simulink model "Controller_20231019"  (R2021b)
settings: Solver=ode4  StartTime=0.0  StopTime=5  FixedStep=0.01  RelTol=1e-3
values from neighbouring files (symbols this model uses):
  diag_M = diagonalize(M_frak0, M_frak)    [Initiate_KUKA_inv.m]
  iota0 = eye(6,6)    [Initiate_KUKA_inv.m]
  K_d = 10*[1.3*eye(3) zeros(3);zeros(3) 0.8*eye(3)]    [Initiate_FQ.m]    (also in Initiate_KUKA_inv.m = 5*[0.7*eye(3) zeros(3);zeros(3) 0.5*eye(3)])
  K_i = 5*[0.1*eye(3) zeros(3);zeros(3) 0.01*eye(3)]    [Initiate_FQ.m]    (also in Initiate_KUKA_inv.m = 5*[0.01*eye(3) zeros(3);zeros(3) 0.001*eye(3)])
  K_p = 100*[0.1 0 0 0 0 0;0 0.1 0 0 0 0; 0 0 0.1 0 0 0; 0 0 0 0.01 0 0 ... (first row only)    [Initiate_FQ.m]    (also in Initiate_KUKA_inv.m = 5*[0.1 0 0 0 0 0;0 0.1 0 0 0 0; 0 0 0.1 0 0 0; 0 0 0 0.01 0 )
  m0 = robot.Bodies{1,n+1}.Mass    [Initiate_KUKA_inv.m]
  M_t = (((Adjoint(g_It))'\M_t_body)/(Adjoint(g_It)))    [Initiate_FQ.m]    (also in Initiate_KUKA_inv.m = [eye(3)*mt zeros(3); zeros(3) eye(3)*80])
  mm = zeros(1,n)    [Initiate_KUKA_inv.m]
  mu = P0    [Initiate_FQ.m]    (also in Initiate_KUKA_inv.m = zeros(6,1))
  mu_t = inv((Adjoint(g_It))')*M_t_body*[V_It;w_t]    [Initiate_FQ.m]    (also in Initiate_KUKA_inv.m = M_t*[V_0t;w_t])
  q_dot_m = [0;0;0;0;0;0;0]    [Initiate_FQ.m]    (also in Initiate_KUKA_inv.m)
  q_m = [0.2;1.2;0.3;2.5;0.5;1.5;0.6]    [Initiate_FQ.m]    (also in Initiate_KUKA_inv.m = [0;0;0;0;0;0;0])
  rho_0t = [0.24;0.26;0.25]    [Initiate_KUKA_inv.m]
  sc_size = 1    [Initiate_KUKA_inv.m]
  V_0t = [-0.01;-0.01;0]    [Initiate_KUKA_inv.m]
  V_I0 = [-0.001;-0.001;0.0;-0.001;0.001;0.002]    [Initiate_FQ.m]    (also in Initiate_KUKA_inv.m = [0;0;0;0;0;0])
  Xi_m_matrix = zeros(6*n,n)    [Initiate_KUKA_inv.m]
undefined symbols (not defined in the file or in its folder): I0, Ie, Im, me, X, Xi_m, Y, Z
libraries: nesl_utility x83, sm_lib x78, robotcorelib x4
(part 1 of 4)
settings Model: Creator=Bmmog  LastModifiedBy=Bmmog

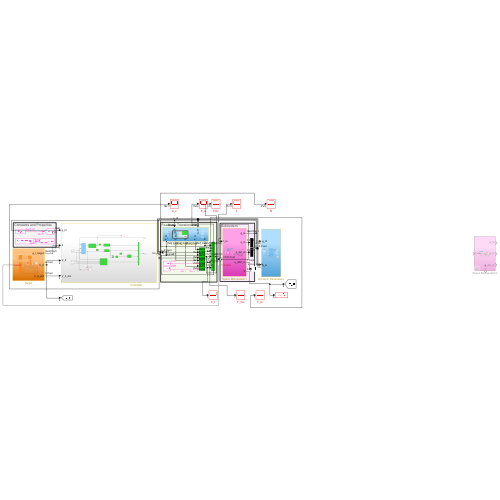
[thumbnail: Simulink's stored preview of the top-level diagram]
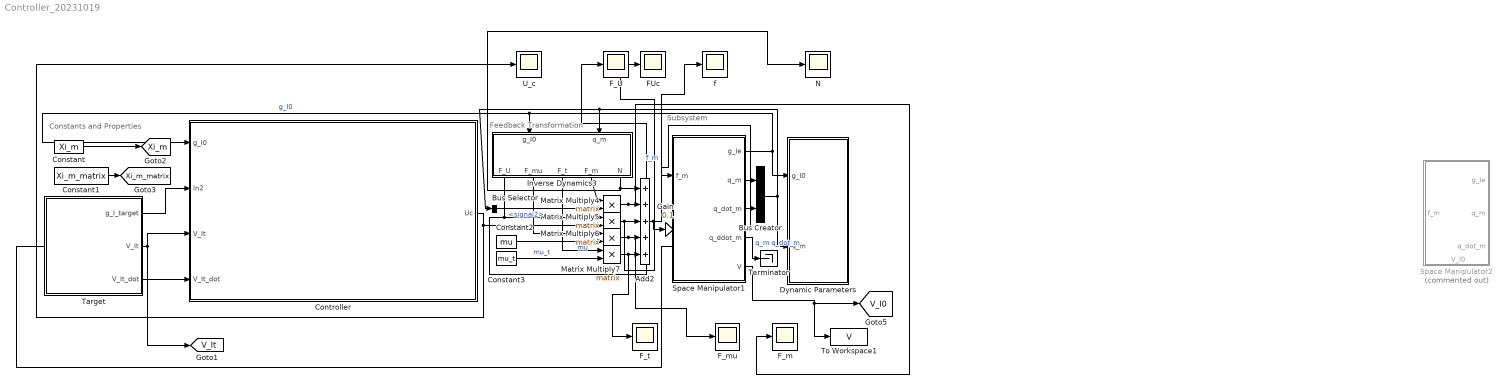
== system Controller_20231019 ==
  note: Subsystem
  note: Constants and Properties
  note: Feedback Transformation
  "\t\t\t\t\t\t\t\t\t\tController" : Subsystem
  Add2 : Sum  Inputs=+++++
  Bus Creator : BusCreator  Inputs=2
  Bus Selector : BusSelector  OutputSignals=signal2
  Constant : Constant  Value=Xi_m
  Constant1 : Constant  Value=Xi_m_matrix
  Constant2 : Constant  Value=mu
  Constant3 : Constant  Value=mu_t
  Dynamic Parameters : Subsystem
  FUc : Scope
  F_U : Scope
  F_m : Scope
  F_mu : Scope
  F_t : Scope
  Gain : Gain  Gain=0.1
  Inverse Dynamics3 : Subsystem
  Matrix Multiply{4..7} (4 alike) : Product  Multiplication=Matrix(*)
  N : Scope
  Space Manipulator1 : Subsystem
  Space Manipulator2 : Subsystem  Commented=on
      settings: PortSchema="{\"entries\":[{\"content\":{\"sides\":[{\"content\":{\"connectorIds\":[\"In1\"]},\"type\":\"ConnectorPlacement.EquallySpacedRectSide\",\"uuid\":\"530c21f8-fd54-4a84-9ce8-3a95f84fd0bc\"},{\"content\":{\"connectorIds\":[\"Out1\",\"Out2\",\"Out3\"],\"side\":\"RIGHT\"},\"type\":\"ConnectorPlacement.EquallySpacedRectSide\",\"uuid\":\"3d1ca3bb-457e-45f0-8a55-d4d08374b273\"},{\"content\":{\"connectorIds\":[],\"side\":\"TOP\"},\"type\":\"ConnectorPlacement.EquallySpacedRectSide\",\"uuid\":\"24d553c5-4913-4f02-8b85-43cdd650a04b\"},{\"content\":{\"connectorIds\":[\"Out4\"],\"side\":\"BOTTOM\"},\"type\":\"ConnectorPlacement.EquallySpacedRectSide\",\"uuid\":\"b0ec554d-8dce-4af2-8e04-261e5fffea9f\"}]},\"type\":\"ConnectorPlacement.EquallySpacedConnector\",\"uuid\":\"032cf2d7-4a61-467d-a02b-78dcb243a1bb\"}],\"packageUris\":[\"http://schema.mathworks.com/mf0/Connector/R2020b\"],\"version\":\"1.0\"}"
  Target : Subsystem
  Terminator : Terminator
  To Workspace1 : ToWorkspace  VariableName=V  SaveFormat=Timeseries  SampleTime=-1
  U_c : Scope
  f : Scope
  tag scope: V_I0=global, V_It=global, Xi_m=global, Xi_m_matrix=global
  wires:
  Constant/1 -> [Xi_m]
  Constant1/1 -> [Xi_m_matrix]
  Target/2(V_It) -> "\t\t\t\t\t\t\t\t\t\tController"/3(V_It), [V_It]
  Space Manipulator1/1(g_Ie) -> Dynamic Parameters/1(g_I0), "\t\t\t\t\t\t\t\t\t\tController"/1(g_I0), Inverse Dynamics3/1(g_I0)  "g_I0"
  Inverse Dynamics3/3(F_t) -> Matrix Multiply7/1
  Add2/1 -> f/1, Gain/1  "f_m"
  Matrix Multiply4/1 -> F_m/1, Add2/2
  Matrix Multiply5/1 -> FUc/1, Add2/3
  Matrix Multiply6/1 -> F_mu/1, Add2/4
  Matrix Multiply7/1 -> F_t/1, Add2/5
  Inverse Dynamics3/2(F_mu) -> Matrix Multiply6/1
  Inverse Dynamics3/4(F_m) -> Matrix Multiply4/1
  Constant3/1 -> Matrix Multiply7/2  "mu_t"
  Constant2/1 -> Matrix Multiply6/2  "mu"
  Space Manipulator1/3(q_dot_m) -> Bus Creator/2
  Bus Creator/1 -> Dynamic Parameters/2(q_m), Bus Selector/1, Inverse Dynamics3/2("q_m ")
  Bus Selector/1 -> Matrix Multiply4/2  "<signal2>"
  Inverse Dynamics3/1(F_U) -> F_U/1, Matrix Multiply5/1
  Inverse Dynamics3/5(N) -> N/1, Add2/1
  Space Manipulator1/2(q_m) -> Bus Creator/1
  Space Manipulator1/5(V) -> [V_I0], To Workspace1/1
  Space Manipulator1/4(q_ddot_m) -> Terminator/1  "q_m q_dot_m"
  Gain/1 -> Space Manipulator1/1(f_m)
  "\t\t\t\t\t\t\t\t\t\tController"/1(Uc) -> U_c/1, Matrix Multiply5/2
  Target/1(g_I_target) -> "\t\t\t\t\t\t\t\t\t\tController"/2(In2)
  Target/3(V_It_dot) -> "\t\t\t\t\t\t\t\t\t\tController"/4(V_It_dot)
  connections:
  Target/LConn1 -- Space Manipulator1/LConn1

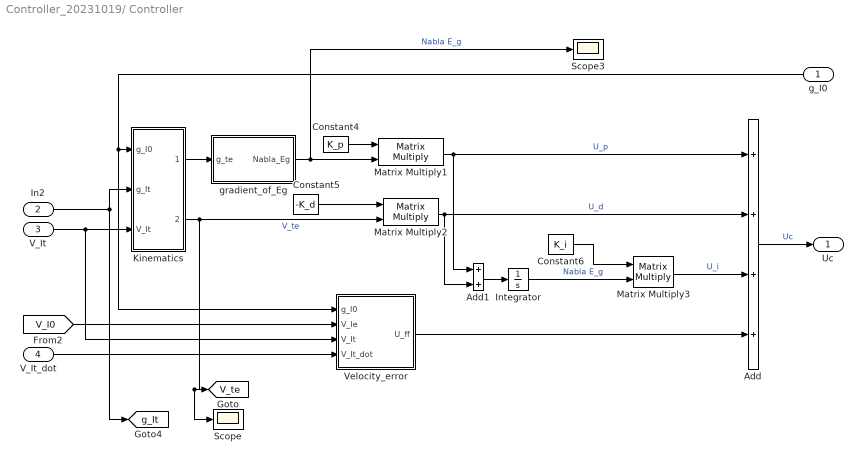
== system Controller_20231019/										Controller ==
  g_I0 : Inport
  In2 : Inport  Port=2
  V_It : Inport  Port=3
  V_It_dot : Inport  Port=4
  Add : Sum  Inputs=++++
  Add1 : Sum
  Constant4 : Constant  Value=K_p
  Constant5 : Constant  Value=-K_d
  Constant6 : Constant  Value=K_i
  Integrator : Integrator
  Kinematics : Subsystem
  Matrix Multiply1 : Product  Multiplication=Matrix(*)
  Matrix Multiply2 : Product  Multiplication=Matrix(*)
  Matrix Multiply3 : Product  Multiplication=Matrix(*)
  Scope : Scope
  Scope3 : Scope
  Velocity_error : MATLAB Function  TreatAsAtomicUnit=on
  gradient_of_Eg : MATLAB Function  TreatAsAtomicUnit=on
  Uc : Outport
  tag scope: V_te=global, g_It=global
  wires:
  Kinematics/2(V_te) -> Matrix Multiply2/2, Scope/1, [V_te]  "V_te"
  In2/1 -> [g_It], Kinematics/2(g_It)
  Add1/1 -> Integrator/1
  Matrix Multiply1/1 -> Add1/1, Add/1  "U_p"
  Constant6/1 -> Matrix Multiply3/1
  Matrix Multiply2/1 -> Add1/2, Add/2  "U_d"
  Integrator/1 -> Matrix Multiply3/2  "Nabla E_g"
  gradient_of_Eg/1(Nabla_Eg) -> Scope3/1, Matrix Multiply1/2  "Nabla E_g"
  Constant4/1 -> Matrix Multiply1/1
  Constant5/1 -> Matrix Multiply2/1
  Kinematics/1(g_te1) -> gradient_of_Eg/1(g_te)
  Matrix Multiply3/1 -> Add/3  "U_i"
  g_I0/1 -> Velocity_error/1(g_I0), Kinematics/1(g_I0)
  Add/1 -> Uc/1  "Uc"
  V_It/1 -> Velocity_error/3(V_It), Kinematics/3(V_It)
  [V_I0] -> Velocity_error/2(V_Ie)
  V_It_dot/1 -> Velocity_error/4(V_It_dot)
  Velocity_error/1(U_ff) -> Add/4

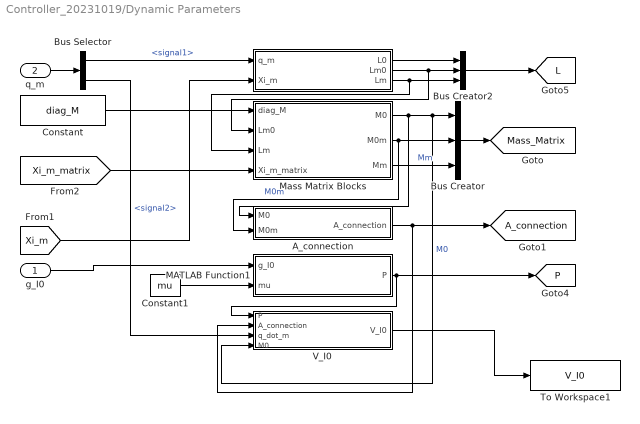
== system Controller_20231019/Dynamic Parameters ==
  g_I0 : Inport
  q_m : Inport  Port=2
  " " : MATLAB Function  TreatAsAtomicUnit=on
  A_connection : Subsystem
  Bus Creator : BusCreator  Inputs=3
  Bus Creator2 : BusCreator  Inputs=3
  Bus Selector : BusSelector  OutputSignals=signal1,signal2
  Constant : Constant  Value=diag_M  VectorParams1D=off
  Constant1 : Constant  Value=mu
  MATLAB Function1 : MATLAB Function  TreatAsAtomicUnit=on
  Mass Matrix Blocks : Subsystem
  To Workspace1 : ToWorkspace  VariableName=V_I0  SaveFormat=Timeseries  SampleTime=-1
  V_I0 : MATLAB Function  TreatAsAtomicUnit=on
  tag scope: A_connection=global, L=global, Mass_Matrix=global, P=global
  wires:
  Mass Matrix Blocks/1(M0) -> V_I0/4(M0), Bus Creator/1, A_connection/1(M0)  "M0"
  Mass Matrix Blocks/2(M0m) -> Bus Creator/2, A_connection/2(M0m)  "M0m"
  Mass Matrix Blocks/3(Mm) -> Bus Creator/3  "Mm"
  Bus Creator/1 -> [Mass_Matrix]
  A_connection/1(A_connection) -> V_I0/2(A_connection), [A_connection]
  V_I0/1(V_I0) -> To Workspace1/1
  MATLAB Function1/1(P) -> [P], V_I0/1(P)
  Constant1/1 -> MATLAB Function1/2(mu)
  q_m/1 -> Bus Selector/1
  g_I0/1 -> MATLAB Function1/1(g_I0)
  [Xi_m] -> " "/2(Xi_m)
  " "/2(Lm0) -> Bus Creator2/2, Mass Matrix Blocks/2(Lm0)
  " "/3(Lm) -> Mass Matrix Blocks/3(Lm), Bus Creator2/3
  Constant/1 -> Mass Matrix Blocks/1(diag_M)
  [Xi_m_matrix] -> Mass Matrix Blocks/4(Xi_m_matrix)
  " "/1(L0) -> Bus Creator2/1
  Bus Creator2/1 -> [L]
  Bus Selector/1 -> " "/1(q_m)  "<signal1>"
  Bus Selector/2 -> V_I0/3(q_dot_m)  "<signal2>"

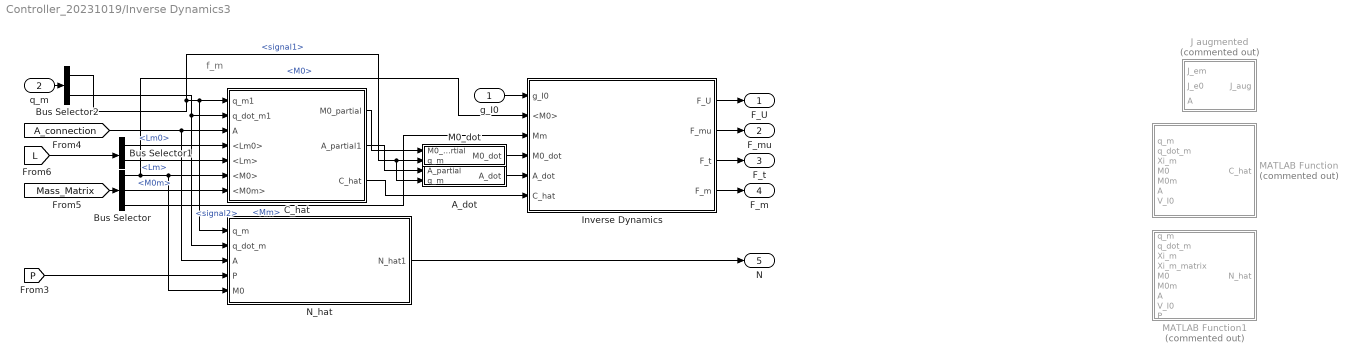
== system Controller_20231019/Inverse Dynamics3 ==
  note: f_m
  g_I0 : Inport
  "q_m " : Inport  Port=2
  A_dot : MATLAB Function  TreatAsAtomicUnit=on
  Bus Selector : BusSelector  OutputSignals=M0,M0m,Mm
  Bus Selector1 : BusSelector  OutputSignals=Lm0,Lm
  Bus Selector2 : BusSelector  OutputSignals=signal1,signal2
  C_hat : Subsystem
  Inverse Dynamics : Subsystem
  J augmented : MATLAB Function  Commented=on  TreatAsAtomicUnit=on
  M0_dot : MATLAB Function  TreatAsAtomicUnit=on
  MATLAB Function : MATLAB Function  Commented=on  TreatAsAtomicUnit=on
  MATLAB Function1 : MATLAB Function  Commented=on  TreatAsAtomicUnit=on
  N_hat : Subsystem
  F_U : Outport
  F_mu : Outport  Port=2
  F_t : Outport  Port=3
  F_m : Outport  Port=4
  N : Outport  Port=5
  wires:
  N_hat/1(N_hat1) -> N/1
  [P] -> N_hat/4(P)
  [Mass_Matrix] -> Bus Selector/1
  Bus Selector/1 -> C_hat/6(<M0>), N_hat/5(M0), Inverse Dynamics/2(<M0>)  "<M0>"
  [L] -> Bus Selector1/1
  g_I0/1 -> Inverse Dynamics/1(g_I0)
  Inverse Dynamics/1(F_U) -> F_U/1
  Inverse Dynamics/2(F_mu) -> F_mu/1
  Inverse Dynamics/3(F_t) -> F_t/1
  Inverse Dynamics/4(F_m) -> F_m/1
  Bus Selector/3 -> Inverse Dynamics/3(Mm)  "<Mm>"
  Bus Selector2/1 -> M0_dot/2(q_m), A_dot/2(q_m), N_hat/1(q_m), C_hat/1(q_m1)  "<signal1>"
  Bus Selector2/2 -> N_hat/2(q_dot_m), C_hat/2(q_dot_m1)  "<signal2>"
  [A_connection] -> C_hat/3(A), N_hat/3(A)
  Bus Selector1/1 -> C_hat/4(<Lm0>)  "<Lm0>"
  Bus Selector1/2 -> C_hat/5(<Lm>)  "<Lm>"
  Bus Selector/2 -> C_hat/7(<M0m>)  "<M0m>"
  C_hat/1(M0_partial) -> M0_dot/1(M0_partial)
  C_hat/2(A_partial1) -> A_dot/1(A_partial)
  C_hat/3(C_hat) -> Inverse Dynamics/6(C_hat)
  M0_dot/1(M0_dot) -> Inverse Dynamics/4(M0_dot)
  A_dot/1(A_dot) -> Inverse Dynamics/5(A_dot)
  "q_m "/1 -> Bus Selector2/1

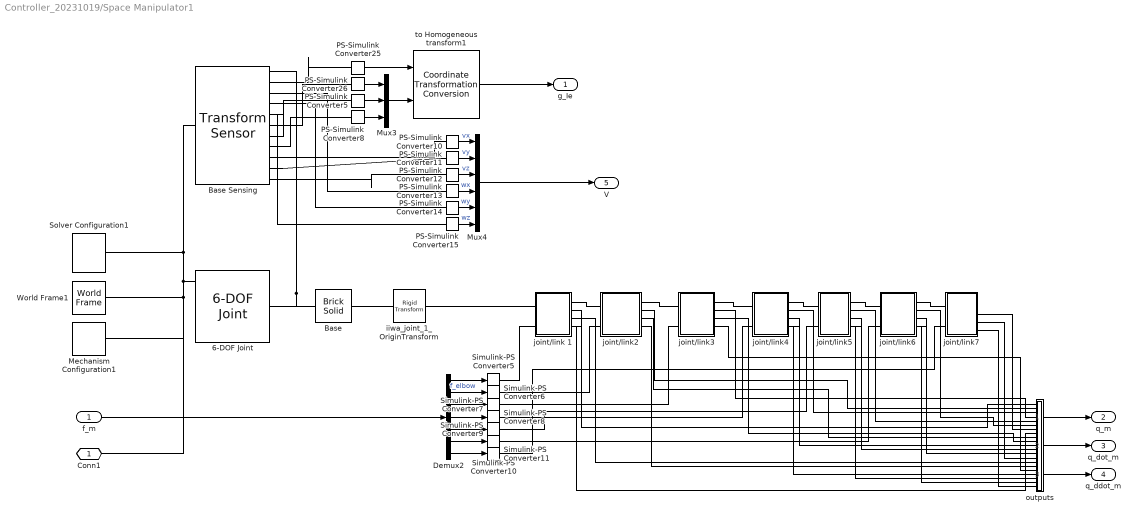
== system Controller_20231019/Space Manipulator1 ==
  f_m : Inport
  6-DOF Joint : sm_lib/Joints/6-DOF Joint  JointMode=Normal  SenseConstraintForce=off  SenseConstraintForceX=off  SenseConstraintForceY=off  SenseConstraintForceZ=off  SenseConstraintTorque=off  SenseConstraintTorqueX=off  SenseConstraintTorqueY=off  SenseConstraintTorqueZ=off  SenseTotalForce=off  SenseTotalForceX=off  SenseTotalForceY=off  SenseTotalForceZ=off  SenseTotalTorque=off  SenseTotalTorqueX=off  SenseTotalTorqueY=off  SenseTotalTorqueZ=off  CompositeWrenchDir=FollowerOnBase  CompositeWrenchFrame=BaseFrame  PxEquilibriumPosition=0  PxEquilibriumPositionUnits=m  PxSpringStiffness=0  PxSpringStiffnessUnits=N/m  PxDampingCoefficient=0  PxDampingCoefficientUnits=N/(m/s)  PxTorqueActuationMode=InputTorque  PxMotionActuationMode=ComputedMotion  PxSensePosition=off  PxSenseVelocity=off  PxSenseAcceleration=off  PxSenseTorqueForce=off  PxSenseLowerLimitTorqueForce=off  PxSenseUpperLimitTorqueForce=off  PxLowerLimitSpecify=off  PxLowerLimitBound=-1  PxLowerLimitBoundUnits=m  PxLowerLimitStiffness=1e6  PxLowerLimitStiffnessUnits=N/m  PxLowerLimitDamping=1e3  PxLowerLimitDampingUnits=N/(m/s)  PxLowerLimitTransitionRegionWidth=1e-4  PxLowerLimitTransitionRegionWidthUnits=m  PxUpperLimitSpecify=off  PxUpperLimitBound=1  PxUpperLimitBoundUnits=m  PxUpperLimitStiffness=1e6  PxUpperLimitStiffnessUnits=N/m  PxUpperLimitDamping=1e3  PxUpperLimitDampingUnits=N/(m/s)  PxUpperLimitTransitionRegionWidth=1e-4  PxUpperLimitTransitionRegionWidthUnits=m  PxPositionTargetSpecify=off  PxPositionTargetPriority=High  PxPositionTargetValue=0  PxPositionTargetValueUnits=m  PxVelocityTargetSpecify=on  PxVelocityTargetPriority=High  PxVelocityTargetValue=V_I0(1)  PxVelocityTargetValueUnits=m/s  PyEquilibriumPosition=0  PyEquilibriumPositionUnits=m  PySpringStiffness=0  PySpringStiffnessUnits=N/m  PyDampingCoefficient=0  PyDampingCoefficientUnits=N/(m/s)  PyTorqueActuationMode=InputTorque  PyMotionActuationMode=ComputedMotion  PySensePosition=off  PySenseVelocity=off  PySenseAcceleration=off  PySenseTorqueForce=off  PySenseLowerLimitTorqueForce=off  PySenseUpperLimitTorqueForce=off  PyLowerLimitSpecify=off  PyLowerLimitBound=-1  PyLowerLimitBoundUnits=m  PyLowerLimitStiffness=1e6  PyLowerLimitStiffnessUnits=N/m  PyLowerLimitDamping=1e3  PyLowerLimitDampingUnits=N/(m/s)  PyLowerLimitTransitionRegionWidth=1e-4  PyLowerLimitTransitionRegionWidthUnits=m  PyUpperLimitSpecify=off  PyUpperLimitBound=1  PyUpperLimitBoundUnits=m  PyUpperLimitStiffness=1e6  PyUpperLimitStiffnessUnits=N/m  PyUpperLimitDamping=1e3  PyUpperLimitDampingUnits=N/(m/s)  PyUpperLimitTransitionRegionWidth=1e-4  PyUpperLimitTransitionRegionWidthUnits=m  PyPositionTargetSpecify=off  PyPositionTargetPriority=High  PyPositionTargetValue=0  PyPositionTargetValueUnits=m  PyVelocityTargetSpecify=on  PyVelocityTargetPriority=High  PyVelocityTargetValue=V_I0(2)  PyVelocityTargetValueUnits=m/s  PzEquilibriumPosition=0  PzEquilibriumPositionUnits=m  PzSpringStiffness=0  PzSpringStiffnessUnits=N/m  PzDampingCoefficient=0  PzDampingCoefficientUnits=N/(m/s)  PzTorqueActuationMode=InputTorque  PzMotionActuationMode=ComputedMotion  PzSensePosition=off  PzSenseVelocity=off  PzSenseAcceleration=off  PzSenseTorqueForce=off  PzSenseLowerLimitTorqueForce=off  PzSenseUpperLimitTorqueForce=off  PzLowerLimitSpecify=off  PzLowerLimitBound=-1  PzLowerLimitBoundUnits=m  PzLowerLimitStiffness=1e6  PzLowerLimitStiffnessUnits=N/m  PzLowerLimitDamping=1e3  PzLowerLimitDampingUnits=N/(m/s)  PzLowerLimitTransitionRegionWidth=1e-4  PzLowerLimitTransitionRegionWidthUnits=m  PzUpperLimitSpecify=off  PzUpperLimitBound=1  PzUpperLimitBoundUnits=m  PzUpperLimitStiffness=1e6  PzUpperLimitStiffnessUnits=N/m  PzUpperLimitDamping=1e3  PzUpperLimitDampingUnits=N/(m/s)  PzUpperLimitTransitionRegionWidth=1e-4  PzUpperLimitTransitionRegionWidthUnits=m  PzPositionTargetSpecify=off  PzPositionTargetPriority=High  PzPositionTargetValue=0  PzPositionTargetValueUnits=m  PzVelocityTargetSpecify=on  PzVelocityTargetPriority=High  PzVelocityTargetValue=V_I0(3)  PzVelocityTargetValueUnits=m/s  SphDefPosRotationMethod=None  SphDefPosRotationAngleUnits=deg  SphDefPosRotationStandardAxis=+Z  SphDefPosRotationAngle=0.0  SphDefPosRotationArbitraryAxis=[0 0 1]  SphDefPosFollAlignAxisA=+X  SphDefPosBaseAlignAxisA=+Y  SphDefPosFollAlignAxisB=+Y  SphDefPosBaseAlignAxisB=+Z  SphDefPosRotationSequenceAxes=FollowerAxes  SphDefPosRotationSequence=XYX  SphDefPosRotationSequenceAngles=[0 0 0]  SphDefPosRotationSequenceAnglesUnits=deg  SphDefPosRotationMatrix=[1 0 0; 0 1 0; 0 0 1]  SphEqPosRotationMethod=None  SphEqPosRotationAngleUnits=deg  SphEqPosRotationStandardAxis=+Z  SphEqPosRotationAngle=0.0  SphEqPosRotationArbitraryAxis=[0 0 1]  SphEqPosFollAlignAxisA=+X  SphEqPosBaseAlignAxisA=+Y  SphEqPosFollAlignAxisB=+Y  SphEqPosBaseAlignAxisB=+Z  SphEqPosRotationSequenceAxes=FollowerAxes  SphEqPosRotationSequence=XYX  SphEqPosRotationSequenceAngles=[0 0 0]  SphEqPosRotationSequenceAnglesUnits=deg  SphEqPosRotationMatrix=[1 0 0; 0 1 0; 0 0 1]  SphSpringStiffness=0  SphSpringStiffnessUnits=N*m/deg  SphDampingCoefficient=0  SphDampingCoefficientUnits=N*m/(deg/s)  SphActuateTorqueX=off  SphActuateTorqueY=off  SphActuateTorqueZ=off  SphActuateTorque=off  SphTorqueActuationMode=NoTorque  SphMotionActuationMode=ComputedMotion  SphActuationFrame=BaseFrame  SphSensePosition=off  SphSenseVelocityX=off  SphSenseVelocityY=off  SphSenseVelocityZ=off  SphSenseVelocity=off  SphSenseAccelerationX=off  SphSenseAccelerationY=off  SphSenseAccelerationZ=off  SphSenseAcceleration=off  SphSenseTorqueX=off  SphSenseTorqueY=off  SphSenseTorqueZ=off  SphSenseTorqueForce=off  SphSenseLowerLimitTorqueMag=off  SphSenseUpperLimitTorqueMag=off  SphSensingFrame=BaseFrame  SphLowerLimitSpecify=off  SphLowerLimitBound=15  SphLowerLimitBoundUnits=deg  SphLowerLimitStiffness=1e4  SphLowerLimitStiffnessUnits=N*m/deg  SphLowerLimitDamping=10  SphLowerLimitDampingUnits=N*m/(deg/s)  SphLowerLimitTransitionRegionWidth=0.1  SphLowerLimitTransitionRegionWidthUnits=deg  SphUpperLimitSpecify=off  SphUpperLimitBound=45  SphUpperLimitBoundUnits=deg  SphUpperLimitStiffness=1e4  SphUpperLimitStiffnessUnits=N*m/deg  SphUpperLimitDamping=10  SphUpperLimitDampingUnits=N*m/(deg/s)  SphUpperLimitTransitionRegionWidth=0.1  SphUpperLimitTransitionRegionWidthUnits=deg  SphPositionTargetRotationMethod=None  SphPositionTargetRotationAngleUnits=deg  SphPositionTargetRotationStandardAxis=+Z  SphPositionTargetRotationAngle=0.0  SphPositionTargetRotationArbitraryAxis=[0 0 1]  SphPositionTargetFollAlignAxisA=+X  SphPositionTargetBaseAlignAxisA=+Y  SphPositionTargetFollAlignAxisB=+Y  SphPositionTargetBaseAlignAxisB=+Z  SphPositionTargetRotationSequenceAxes=FollowerAxes  SphPositionTargetRotationSequence=XYX  SphPositionTargetRotationSequenceAngles=[0 0 0]  SphPositionTargetRotationSequenceAnglesUnits=deg  SphPositionTargetRotationMatrix=[1 0 0; 0 1 0; 0 0 1]  SphPositionTargetSpecify=off  SphPositionTargetPriority=High  SphVelocityTargetValue=[V_I0(4) V_I0(5) V_I0(6)]  SphVelocityTargetValueUnits=rad/s  SphVelocityTargetSpecify=on  SphVelocityTargetPriority=High  SphVelocityTargetInFollowerFrame=on
  Base : sm_lib/Body Elements/Brick Solid  GraphicAmbientColor=[0.15 0.15 0.15 1.0]  BasedOnType=Mass  BrickDimensions=[sc_size, sc_size, sc_size]  BrickDimensionUnits=m  CenterOfMass=[0 0 0]  CenterOfMassUnits=m  GraphicDiffuseColor=[0.5 0.5 0.5]  Density=1000  DensityUnits=kg/m^3  DoExposeReferenceFrame=on  GraphicEmissiveColor=[0.0 0.0 0.0 1.0]  ExportEntireGeometry=off  SerializedFrames=<Frames><Frame><Id>Frame1</Id><Value><Name>F1</Name><Origin><Source>GeometricFeature</Source><FeatureName>+z surface</FeatureName></Origin><PrimaryAxis><DefinedDirection>+X</DefinedDirection><Source>ReferenceFrame</Source><SourceDirection>+X</SourceDirection><FeatureName></FeatureName></PrimaryAxis><SecondaryAxis><DefinedDirection>+Z</DefinedDirection><Source>ReferenceFrame</Source><SourceDirection>+Z</SourceDirection><FeatureName></FeatureName></SecondaryAxis></Value></Frame></Frames>  MarkerShape=Sphere  MarkerSize=10  GraphicType=FromGeometry  InertiaType=CalculateFromGeometry  Mass=m0  MassUnits=kg  MomentsOfInertia=[I0(1,1) I0(2,2) I0(3,3)]  MomentsOfInertiaUnits=kg*m^2  GraphicOpacity=1.0  ProductsOfInertia=[0 0 0]  ProductsOfInertiaUnits=kg*m^2  GraphicShininess=75  GraphicSpecularColor=[0.5 0.5 0.5 1.0]  GraphicVisPropType=SimpleVisualProperties
  Base Sensing : sm_lib/Frames and Transforms/Transform Sensor  MeasurementFrame=Base  SenseAngle=off  SenseAxis=off  SenseAngle1=off  SenseAngle2=off  SenseAngle3=off  SenseQ=off  SenseR=on  SenseOmegaX=on  SenseOmegaY=on  SenseOmegaZ=on  SenseOmega1=off  SenseOmega2=off  SenseOmega3=off  SenseQDot=off  SenseRDot=off  SenseAlphaX=off  SenseAlphaY=off  SenseAlphaZ=off  SenseAlpha1=off  SenseAlpha2=off  SenseAlpha3=off  SenseQDDot=off  SenseRDDot=off  SenseX=on  SenseY=on  SenseZ=on  SenseRad=off  SenseAzim=off  SenseDist=off  SenseInc=off  SenseXDot=on  SenseYDot=on  SenseZDot=on  SenseRadDot=off  SenseAzimDot=off  SenseDistDot=off  SenseIncDot=off  SenseXDDot=off  SenseYDDot=off  SenseZDDot=off  SenseRadDDot=off  SenseAzimDDot=off  SenseDistDDot=off  SenseIncDDot=off
  Demux2 : Demux  Outputs=7
  Mechanism Configuration1 : sm_lib/Utilities/Mechanism Configuration  UniformGravity=Constant  GravityVector=[0 0 0]  GravityUnits=m/s^2  LinearizationDelta=0.001  JointModeTransitionNonlinearIterations=2
  Mux3 : Mux  Inputs=3
  Mux4 : Mux  Inputs=6
  PS-Simulink Converter{5,8,10..15,25..26} (10 alike) : nesl_utility/PS-Simulink Converter  PhysicalDomain=network_engine_domain  SubClassName=ps_output  LeftPortType=input  RightPortType=output  PseudoPeriodic=off  Frequencies=[]  Unit=inherit  AffineConversion=off
      settings: SourceProductBaseCode=PW,SS
  Simulink-PS Converter{5..11} (7 alike) : nesl_utility/Simulink-PS Converter  PhysicalDomain=network_engine_domain  SubClassName=ps_input  LeftPortType=input  RightPortType=output  PseudoPeriodic=off  Frequencies=[]  NoiseDistribution=none  NoiseParameters=[]  Unit=1  AffineConversion=off  FilteringAndDerivatives=provide  SimscapeFilterOrder=1  InputFilterTimeConstant=0.001  UdotUserProvided=0
      settings: SourceProductBaseCode=PW,SS
  Solver Configuration1 : nesl_utility/Solver Configuration  PhysicalDomain=network_engine_domain  SubClassName=solver  LeftPortType=input  RightPortType=generic  Tones=[]  Harmonics=[]  SimulateNoise=off  Profile=off  UseLocalSampling=off  EnableSwitchedLinearOptims=on  FrequencyDomain=off  UseCCode=off  RelTol=0.001  AbsTol=1e-06  MinStep=1e-09  ToWorkspace=off  RevertToSquareIcSolve=off  NumHomotopyIterations=100  PhasorMode=off  PhasorModeNumHarmonics=1  DoDC=off  ResidualTolerance=1e-09  UseLocalSolver=off  LocalSolverChoice=NE_BACKWARD_EULER_ADVANCER  LocalSolverSampleTime=0.001  DoFixedCost=off  MaxNonlinIter=3  MaxModeIter=2  ComputeImpulses=off  ImpulseIterations=2  LinearAlgebra=Sparse  EquationFormulation=NE_TIME_EF  DelaysMemoryBudget=1024  AutomaticFiltering=on  FilteringTimeConstant=0.001  PartitionStorageMethod=AS_NEEDED  PartitionMemoryBudget=1024  PartitionMethod=FAST
      settings: SourceProductBaseCode=PW,SS
  World Frame1 : sm_lib/Frames and Transforms/World Frame
  iiwa_joint_1_OriginTransform : sm_lib/Frames and Transforms/Rigid Transform  TranslationMethod=Cartesian  TranslationStandardOffset=0  TranslationLengthUnit=m  TranslationStandardAxis=+Z  TranslationCartesianOffset=[0, 0, 0]  TranslationROffset=0  TranslationROffsetUnits=m  TranslationZOffset=0  TranslationZOffsetUnits=m  TranslationThetaOffset=0  TranslationThetaOffsetUnits=deg  RotationMethod=RotationSequence  RotationAngleUnits=deg  RotationStandardAxis=+Z  RotationAngle=0.0  RotationArbitraryAxis=[0 0 1]  FollAlignAxisA=+X  BaseAlignAxisA=+Y  FollAlignAxisB=+Y  BaseAlignAxisB=+Z  RotationSequenceAxes=BaseAxes  RotationSequence=XYZ  RotationSequenceAngles=[0, 0, 0]  RotationSequenceAnglesUnits=rad  RotationMatrix=[1 0 0; 0 1 0; 0 0 1]
  joint/link 1 : Subsystem
  joint/link2 : Subsystem
  joint/link3 : Subsystem
  joint/link4 : Subsystem
  joint/link5 : Subsystem
  joint/link6 : Subsystem
  joint/link7 : Subsystem
  outputs : Subsystem
  to Homogeneous transform1 : robotcorelib/Coordinate Transformation Conversion  InputRepresentation=Rotation Matrix  InputEulerSequence=ZYX  ShowTrVecInputPort=on  OutputRepresentation=Homogeneous Transformation  OutputEulerSequence=ZYX  ShowTrVecOutputPort=on  SimulateUsing=Interpreted execution
      settings: SourceProductBaseCode=NV,RO,RR,UV
  Conn1 : PMIOPort  Side=Left
  g_Ie : Outport
  q_m : Outport  Port=2
  q_dot_m : Outport  Port=3
  q_ddot_m : Outport  Port=4
  V : Outport  Port=5
  wires:
  PS-Simulink Converter25/1 -> to Homogeneous transform1/1
  to Homogeneous transform1/1 -> g_Ie/1
  PS-Simulink Converter5/1 -> Mux3/2
  PS-Simulink Converter8/1 -> Mux3/3
  PS-Simulink Converter26/1 -> Mux3/1
  Mux3/1 -> to Homogeneous transform1/2
  Demux2/1 -> Simulink-PS Converter5/1
  Demux2/6 -> Simulink-PS Converter10/1
  Demux2/3 -> Simulink-PS Converter7/1
  Demux2/2 -> Simulink-PS Converter6/1  "f_elbow"
  Demux2/5 -> Simulink-PS Converter9/1
  Demux2/7 -> Simulink-PS Converter11/1
  outputs/3(q_ddot_m) -> q_ddot_m/1
  f_m/1 -> Demux2/1
  Demux2/4 -> Simulink-PS Converter8/1
  outputs/2(q_dot_m) -> q_dot_m/1
  outputs/1(q_m) -> q_m/1
  PS-Simulink Converter13/1 -> Mux4/4  "wx"
  PS-Simulink Converter12/1 -> Mux4/3  "vz"
  PS-Simulink Converter10/1 -> Mux4/1  "vx"
  Mux4/1 -> V/1
  PS-Simulink Converter11/1 -> Mux4/2  "vy"
  PS-Simulink Converter14/1 -> Mux4/5  "wy"
  PS-Simulink Converter15/1 -> Mux4/6  "wz"
  connections:
  Base Sensing/LConn1 -- Conn1/RConn1 -- Mechanism Configuration1/RConn1 -- World Frame1/RConn1 -- 6-DOF Joint/LConn1 -- Solver Configuration1/RConn1
  Base Sensing/RConn1 -- Base/RConn1 -- 6-DOF Joint/RConn1
  Base Sensing/RConn6 -- PS-Simulink Converter26/LConn1
  Base Sensing/RConn8 -- PS-Simulink Converter8/LConn1
  Base Sensing/RConn2 -- PS-Simulink Converter25/LConn1
  Base Sensing/RConn7 -- PS-Simulink Converter5/LConn1
  iiwa_joint_1_OriginTransform/RConn1 -- joint/link 1/LConn1
  joint/link3/RConn3 -- outputs/LConn10
  joint/link5/RConn3 -- outputs/LConn12
  Simulink-PS Converter9/RConn1 -- joint/link5/LConn2
  joint/link4/LConn1 -- joint/link3/RConn1
  joint/link4/RConn3 -- outputs/LConn11
  joint/link5/RConn4 -- outputs/LConn19
  Simulink-PS Converter10/RConn1 -- joint/link6/LConn2
  joint/link5/LConn1 -- joint/link4/RConn1
  joint/link7/RConn5 -- outputs/LConn21
  joint/link2/RConn4 -- outputs/LConn16
  joint/link 1/LConn2 -- Simulink-PS Converter5/RConn1
  outputs/LConn1 -- joint/link 1/RConn2
  joint/link5/RConn2 -- outputs/LConn5
  joint/link7/RConn3 -- outputs/LConn7
  joint/link7/RConn4 -- outputs/LConn14
  joint/link2/RConn2 -- outputs/LConn2
  Simulink-PS Converter11/RConn1 -- joint/link7/LConn2
  joint/link 1/RConn3 -- outputs/LConn8
  Simulink-PS Converter7/RConn1 -- joint/link3/LConn2
  joint/link6/LConn1 -- joint/link5/RConn1
  joint/link2/RConn3 -- outputs/LConn9
  joint/link 1/RConn4 -- outputs/LConn15
  Simulink-PS Converter6/RConn1 -- joint/link2/LConn2
  joint/link3/LConn1 -- joint/link2/RConn1
  joint/link4/RConn2 -- outputs/LConn4
  joint/link6/RConn2 -- outputs/LConn6
  joint/link4/RConn4 -- outputs/LConn18
  joint/link3/RConn2 -- outputs/LConn3
  joint/link6/RConn3 -- outputs/LConn13
  Simulink-PS Converter8/RConn1 -- joint/link4/LConn2
  joint/link6/RConn4 -- outputs/LConn20
  joint/link3/RConn4 -- outputs/LConn17
  joint/link7/LConn1 -- joint/link6/RConn1
  joint/link 1/RConn1 -- joint/link2/LConn1
  Base/LConn1 -- iiwa_joint_1_OriginTransform/LConn1
  Base Sensing/RConn9 -- PS-Simulink Converter10/LConn1
  Base Sensing/RConn10 -- PS-Simulink Converter11/LConn1
  Base Sensing/RConn11 -- PS-Simulink Converter12/LConn1
  Base Sensing/RConn3 -- PS-Simulink Converter13/LConn1
  Base Sensing/RConn4 -- PS-Simulink Converter14/LConn1
  Base Sensing/RConn5 -- PS-Simulink Converter15/LConn1
